simulink model "LGS_allFaultsSelected"  (R2019b)
settings: Solver=FixedStepDiscrete  StartTime=0.0  StopTime=45.0  FixedStep=0.1  RelTol=1e-3
model workspace (MAT data in the model file):
  fipData : object (value not decoded)
  fipName : object (value not decoded)
  stepSize = 0.1
undefined symbols (not defined in the file): ActualSystemCondition, ExpectedSystemBehavior, FailureCondition, FailureConditionObserver, LibFailureCondition
libraries: LibFaultInjectionControls x190, commrandsrc3 x70, simulink x3
(part 15 of 41)

== system LGS_allFaultsSelected/Doors/right door zylinder/sensor open/FIP1 ==
  In1 : Inport
  RD sensor open FIP1 : Subsystem  mask(FailureInjectionPoint){}
      mask help: FailureInjectionPoint
      mask init: same as LGS_allFaultsSelected/Analogical switch and general electro-valve and pressure sensor/Analogical switch/Analog Switch FIP
      settings: OpenFcn=|
      | open_system(gcb,'mask');
      | 
      | treeValues = FailureInjectionPointHelper.getAllFmAndParamsAsTreeString(gcb);
      | mo = Simulink.Mask.get(gcb);
      | dc = mo.getDialogControl('GbFmInfo');
      | treeView = dc.getDialogControl('TreeViewFM');
      | treeView.TreeItems = {};
      | treeView.TreeItems = treeValues;
      mask Help: FailureInjectionPoint
      mask DialogControl Control7 Prompt: Containing Failure Modes
      mask DialogControl BtnMoveUp Prompt: Move up
      mask DialogControl BtnMoveUp Callback:
      | %Get name of the failure mode block
      | mo = Simulink.Mask.get(gcb);
      | dc = mo.getDialogControl('GbFmInfo');
      | treeView = dc.getDialogControl('TreeViewFM');
      | try
      |     a = treeView.getSelectedItems();
      |     p = split(a, '/'); %name of failure mode block is p{1}
      | catch
      |     return;
      | end
      | 
      | %Save port handles
      | lh = get_param([gcb,'/',p{1}],'LineHandles');
      | ph = get_param([gcb,'/',p{1}],'PortHandles');
      | this_in = ph.Inport(1);
      | this_out = ph.Outport(1);
      | 
      | last_block = get_param(lh.Inport(1),'SrcBlockHandle');
      | last_block_type = get_param(last_block,'BlockType');
      | if strcmp(last_block_type,'Inport')
      |     return;
      | end
      | lb_lh = get_param(last_block,'LineHandles');
      | 
      | last_out = get_param(lh.Inport(1),'SrcPortHandle');
      | last_in = get_param(lb_lh.Inport(1),'DstPortHandle');
      | next_to_last_out = get_param(lb_lh.Inport(1),'SrcPortHandle');
      | next_in = get_param(lh.Outport(1),'DstPortHandle');
      | 
      | %Delete connecting lines
      | delete_line(lh.Inport(1));
      | delete_line(lh.Outport(1));
      | delete_line(lb_lh.Inport(1));
      | 
      | % Generate new lines
      | add_line(gcb, last_out, next_in, 'autorouting', 'smart');
      | add_line(gcb, this_out, last_in, 'autorouting', 'smart');
      | add_line(gcb, next_to_last_out, this_in, 'autorouting', 'smart');
      | 
      | %Rearrange system
      | Simulink.BlockDiagram.arrangeSystem(gcb);
      | 
      | %Refresh
      | treeValues = FailureInjectionPointHelper.getAllFmAndParamsAsTreeString(gcb);
      | mo = Simulink.Mask.get(gcb);
      | dc = mo.getDialogControl('GbFmInfo');
      | treeView = dc.getDialogControl('TreeViewFM');
      | treeView.TreeItems = {};
      | treeView.TreeItems = treeValues;
      mask DialogControl BtnMoveDown Prompt: Move down
      mask DialogControl BtnMoveDown Callback:
      | %Get name of the failure mode block
      | mo = Simulink.Mask.get(gcb);
      | dc = mo.getDialogControl('GbFmInfo');
      | treeView = dc.getDialogControl('TreeViewFM');
      | try
      |     a = treeView.getSelectedItems();
      |     p = split(a, '/'); %name of failure mode block is p{1}
      | catch
      |     return;
      | end
      | 
      | %Save port handles
      | lh = get_param([gcb,'/',p{1}],'LineHandles');
      | ph = get_param([gcb,'/',p{1}],'PortHandles');
      | this_in = ph.Inport(1);
      | this_out = ph.Outport(1);
      | 
      | next_block = get_param(lh.Outport(1),'DstBlockHandle');
      | next_block_type = get_param(next_block,'BlockType');
      | if strcmp(next_block_type,'Outport')
      |     return;
      | end
      | nb_lh = get_param(next_block,'LineHandles');
      | 
      | last_out = get_param(lh.Inport(1),'SrcPortHandle');
      | next_out = get_param(nb_lh.Outport(1),'SrcPortHandle');
      | next_but_one_in = get_param(nb_lh.Outport(1),'DstPortHandle');
      | next_in = get_param(lh.Outport(1),'DstPortHandle');
      | 
      | %Delete connecting lines
      | delete_line(lh.Inport(1));
      | delete_line(lh.Outport(1));
      | delete_line(nb_lh.Outport(1));
      | 
      | % Generate new lines
      | add_line(gcb, last_out, next_in, 'autorouting', 'smart');
      | add_line(gcb, next_out, this_in, 'autorouting', 'smart');
      | add_line(gcb, this_out, next_but_one_in, 'autorouting', 'smart');
      | 
      | %Rearrange system
      | Simulink.BlockDiagram.arrangeSystem(gcb);
      | 
      | %Refresh
      | treeValues = FailureInjectionPointHelper.getAllFmAndParamsAsTreeString(gcb);
      | mo = Simulink.Mask.get(gcb);
      | dc = mo.getDialogControl('GbFmInfo');
      | treeView = dc.getDialogControl('TreeViewFM');
      | treeView.TreeItems = {};
      | treeView.TreeItems = treeValues;
      mask DialogControl TreeViewFM Prompt: Failure Mode Information
      mask DialogControl BtnOpen Prompt: Open FIP
      mask DialogControl BtnOpen Callback: open_system(gcb,'force');
      mask DialogControl BtnNew Prompt: New
      mask DialogControl BtnNew Callback:
      | dialog_fipManager_single(gcb, '');
      | 
      | %Enable move, edit, delete buttons
      | mo = Simulink.Mask.get(gcb);
      | mo.getDialogControl('BtnMoveUp').Enabled = 'on';
      | mo.getDialogControl('BtnMoveDown').Enabled = 'on';
      | mo.getDialogControl('BtnEdit').Enabled = 'on';
      | mo.getDialogControl('BtnDelete').Enabled = 'on';
      mask DialogControl BtnEdit Prompt: Edit
      mask DialogControl BtnEdit Callback:
      | mo = Simulink.Mask.get(gcb);
      | dc = mo.getDialogControl('GbFmInfo');
      | treeView = dc.getDialogControl('TreeViewFM');
      | try
      |     a = treeView.getSelectedItems();
      |     p = split(a, '/');
      | catch
      |     return;
      | end
      | dialog_fipManager_single(gcb, p{1});
      mask DialogControl BtnDelete Prompt: Delete
      mask DialogControl BtnDelete Callback:
      | %Get name of the failure mode block
      | mo = Simulink.Mask.get(gcb);
      | dc = mo.getDialogControl('GbFmInfo');
      | treeView = dc.getDialogControl('TreeViewFM');
      | try
      |     a = treeView.getSelectedItems();
      |     p = split(a, '/'); %name of failure mode block is p{1}
      | catch
      |     return;
      | end
      | 
      | %Save outport handle of the last and inport handle of the next block
      | lh = get_param([gcb,'/',p{1}],'LineHandles');
      | last_out = get_param(lh.Inport(1),'SrcPortHandle');
      | next_in = get_param(lh.Outport(1),'DstPortHandle');
      | 
      | %Delete connecting lines and failure mode block
      | delete_line(lh.Inport(1));
      | delete_line(lh.Outport(1));
      | fm_handle = get_param([gcb,'/',p{1}],'Handle');
      | delete_block(fm_handle);
      | 
      | % Generate new line from outport last to inport next
      | add_line(gcb, last_out, next_in, 'autorouting', 'smart');
      | 
      | %Rearrange system
      | Simulink.BlockDiagram.arrangeSystem(gcb);
      | 
      | %Disable move, edit, delete buttons in case all FMs are deleted
      | last_block = get_param(last_out,'Parent');
      | last_is_inport = strcmp(get_param(last_block,'BlockType'),'Inport');
      | next_block = get_param(next_in,'Parent');
      | next_is_outport = strcmp(get_param(next_block,'BlockType'),'Outport');
      | if (last_is_inport && next_is_outport)
      |     mo.getDialogControl('BtnMoveUp').Enabled = 'off';
      |     mo.getDialogControl('BtnMoveDown').Enabled = 'off';
      |     mo.getDialogControl('BtnEdit').Enabled = 'off';
      |     mo.getDialogControl('BtnDelete').Enabled = 'off';
      | end
      | 
      | %Refresh
      | treeValues = FailureInjectionPointHelper.getAllFmAndParamsAsTreeString(gcb);
      | mo = Simulink.Mask.get(gcb);
      | dc = mo.getDialogControl('GbFmInfo');
      | treeView = dc.getDialogControl('TreeViewFM');
      | treeView.TreeItems = {};
      | treeView.TreeItems = treeValues;
      mask DialogControl BtnRefresh Prompt: Refresh
      mask DialogControl BtnRefresh Callback:
      | set_param(gcb,'LinkStatus','none');
      | 
      | treeValues = FailureInjectionPointHelper.getAllFmAndParamsAsTreeString(gcb);
      | mo = Simulink.Mask.get(gcb);
      | dc = mo.getDialogControl('GbFmInfo');
      | treeView = dc.getDialogControl('TreeViewFM');
      | treeView.TreeItems = {};
      | treeView.TreeItems = treeValues;
      mask Display: image('icons/failure_injection_point.png','center')
  Out1 : Outport
  wires:
  In1/1 -> RD sensor open FIP1/1(In1)
  RD sensor open FIP1/1(Out1) -> Out1/1

== system LGS_allFaultsSelected/Doors/right door zylinder/sensor open/FIP2 ==
  In1 : Inport
  RD sensor open FIP2 : Subsystem  mask(FailureInjectionPoint){}
      mask help: FailureInjectionPoint
      mask init: same as LGS_allFaultsSelected/Analogical switch and general electro-valve and pressure sensor/Analogical switch/Analog Switch FIP
      settings: OpenFcn=|
      | open_system(gcb,'mask');
      | 
      | treeValues = FailureInjectionPointHelper.getAllFmAndParamsAsTreeString(gcb);
      | mo = Simulink.Mask.get(gcb);
      | dc = mo.getDialogControl('GbFmInfo');
      | treeView = dc.getDialogControl('TreeViewFM');
      | treeView.TreeItems = {};
      | treeView.TreeItems = treeValues;
      mask Help: FailureInjectionPoint
      mask DialogControl Control7 Prompt: Containing Failure Modes
      mask DialogControl BtnMoveUp Prompt: Move up
      mask DialogControl BtnMoveUp Callback:
      | %Get name of the failure mode block
      | mo = Simulink.Mask.get(gcb);
      | dc = mo.getDialogControl('GbFmInfo');
      | treeView = dc.getDialogControl('TreeViewFM');
      | try
      |     a = treeView.getSelectedItems();
      |     p = split(a, '/'); %name of failure mode block is p{1}
      | catch
      |     return;
      | end
      | 
      | %Save port handles
      | lh = get_param([gcb,'/',p{1}],'LineHandles');
      | ph = get_param([gcb,'/',p{1}],'PortHandles');
      | this_in = ph.Inport(1);
      | this_out = ph.Outport(1);
      | 
      | last_block = get_param(lh.Inport(1),'SrcBlockHandle');
      | last_block_type = get_param(last_block,'BlockType');
      | if strcmp(last_block_type,'Inport')
      |     return;
      | end
      | lb_lh = get_param(last_block,'LineHandles');
      | 
      | last_out = get_param(lh.Inport(1),'SrcPortHandle');
      | last_in = get_param(lb_lh.Inport(1),'DstPortHandle');
      | next_to_last_out = get_param(lb_lh.Inport(1),'SrcPortHandle');
      | next_in = get_param(lh.Outport(1),'DstPortHandle');
      | 
      | %Delete connecting lines
      | delete_line(lh.Inport(1));
      | delete_line(lh.Outport(1));
      | delete_line(lb_lh.Inport(1));
      | 
      | % Generate new lines
      | add_line(gcb, last_out, next_in, 'autorouting', 'smart');
      | add_line(gcb, this_out, last_in, 'autorouting', 'smart');
      | add_line(gcb, next_to_last_out, this_in, 'autorouting', 'smart');
      | 
      | %Rearrange system
      | Simulink.BlockDiagram.arrangeSystem(gcb);
      | 
      | %Refresh
      | treeValues = FailureInjectionPointHelper.getAllFmAndParamsAsTreeString(gcb);
      | mo = Simulink.Mask.get(gcb);
      | dc = mo.getDialogControl('GbFmInfo');
      | treeView = dc.getDialogControl('TreeViewFM');
      | treeView.TreeItems = {};
      | treeView.TreeItems = treeValues;
      mask DialogControl BtnMoveDown Prompt: Move down
      mask DialogControl BtnMoveDown Callback:
      | %Get name of the failure mode block
      | mo = Simulink.Mask.get(gcb);
      | dc = mo.getDialogControl('GbFmInfo');
      | treeView = dc.getDialogControl('TreeViewFM');
      | try
      |     a = treeView.getSelectedItems();
      |     p = split(a, '/'); %name of failure mode block is p{1}
      | catch
      |     return;
      | end
      | 
      | %Save port handles
      | lh = get_param([gcb,'/',p{1}],'LineHandles');
      | ph = get_param([gcb,'/',p{1}],'PortHandles');
      | this_in = ph.Inport(1);
      | this_out = ph.Outport(1);
      | 
      | next_block = get_param(lh.Outport(1),'DstBlockHandle');
      | next_block_type = get_param(next_block,'BlockType');
      | if strcmp(next_block_type,'Outport')
      |     return;
      | end
      | nb_lh = get_param(next_block,'LineHandles');
      | 
      | last_out = get_param(lh.Inport(1),'SrcPortHandle');
      | next_out = get_param(nb_lh.Outport(1),'SrcPortHandle');
      | next_but_one_in = get_param(nb_lh.Outport(1),'DstPortHandle');
      | next_in = get_param(lh.Outport(1),'DstPortHandle');
      | 
      | %Delete connecting lines
      | delete_line(lh.Inport(1));
      | delete_line(lh.Outport(1));
      | delete_line(nb_lh.Outport(1));
      | 
      | % Generate new lines
      | add_line(gcb, last_out, next_in, 'autorouting', 'smart');
      | add_line(gcb, next_out, this_in, 'autorouting', 'smart');
      | add_line(gcb, this_out, next_but_one_in, 'autorouting', 'smart');
      | 
      | %Rearrange system
      | Simulink.BlockDiagram.arrangeSystem(gcb);
      | 
      | %Refresh
      | treeValues = FailureInjectionPointHelper.getAllFmAndParamsAsTreeString(gcb);
      | mo = Simulink.Mask.get(gcb);
      | dc = mo.getDialogControl('GbFmInfo');
      | treeView = dc.getDialogControl('TreeViewFM');
      | treeView.TreeItems = {};
      | treeView.TreeItems = treeValues;
      mask DialogControl TreeViewFM Prompt: Failure Mode Information
      mask DialogControl BtnOpen Prompt: Open FIP
      mask DialogControl BtnOpen Callback: open_system(gcb,'force');
      mask DialogControl BtnNew Prompt: New
      mask DialogControl BtnNew Callback:
      | dialog_fipManager_single(gcb, '');
      | 
      | %Enable move, edit, delete buttons
      | mo = Simulink.Mask.get(gcb);
      | mo.getDialogControl('BtnMoveUp').Enabled = 'on';
      | mo.getDialogControl('BtnMoveDown').Enabled = 'on';
      | mo.getDialogControl('BtnEdit').Enabled = 'on';
      | mo.getDialogControl('BtnDelete').Enabled = 'on';
      mask DialogControl BtnEdit Prompt: Edit
      mask DialogControl BtnEdit Callback:
      | mo = Simulink.Mask.get(gcb);
      | dc = mo.getDialogControl('GbFmInfo');
      | treeView = dc.getDialogControl('TreeViewFM');
      | try
      |     a = treeView.getSelectedItems();
      |     p = split(a, '/');
      | catch
      |     return;
      | end
      | dialog_fipManager_single(gcb, p{1});
      mask DialogControl BtnDelete Prompt: Delete
      mask DialogControl BtnDelete Callback:
      | %Get name of the failure mode block
      | mo = Simulink.Mask.get(gcb);
      | dc = mo.getDialogControl('GbFmInfo');
      | treeView = dc.getDialogControl('TreeViewFM');
      | try
      |     a = treeView.getSelectedItems();
      |     p = split(a, '/'); %name of failure mode block is p{1}
      | catch
      |     return;
      | end
      | 
      | %Save outport handle of the last and inport handle of the next block
      | lh = get_param([gcb,'/',p{1}],'LineHandles');
      | last_out = get_param(lh.Inport(1),'SrcPortHandle');
      | next_in = get_param(lh.Outport(1),'DstPortHandle');
      | 
      | %Delete connecting lines and failure mode block
      | delete_line(lh.Inport(1));
      | delete_line(lh.Outport(1));
      | fm_handle = get_param([gcb,'/',p{1}],'Handle');
      | delete_block(fm_handle);
      | 
      | % Generate new line from outport last to inport next
      | add_line(gcb, last_out, next_in, 'autorouting', 'smart');
      | 
      | %Rearrange system
      | Simulink.BlockDiagram.arrangeSystem(gcb);
      | 
      | %Disable move, edit, delete buttons in case all FMs are deleted
      | last_block = get_param(last_out,'Parent');
      | last_is_inport = strcmp(get_param(last_block,'BlockType'),'Inport');
      | next_block = get_param(next_in,'Parent');
      | next_is_outport = strcmp(get_param(next_block,'BlockType'),'Outport');
      | if (last_is_inport && next_is_outport)
      |     mo.getDialogControl('BtnMoveUp').Enabled = 'off';
      |     mo.getDialogControl('BtnMoveDown').Enabled = 'off';
      |     mo.getDialogControl('BtnEdit').Enabled = 'off';
      |     mo.getDialogControl('BtnDelete').Enabled = 'off';
      | end
      | 
      | %Refresh
      | treeValues = FailureInjectionPointHelper.getAllFmAndParamsAsTreeString(gcb);
      | mo = Simulink.Mask.get(gcb);
      | dc = mo.getDialogControl('GbFmInfo');
      | treeView = dc.getDialogControl('TreeViewFM');
      | treeView.TreeItems = {};
      | treeView.TreeItems = treeValues;
      mask DialogControl BtnRefresh Prompt: Refresh
      mask DialogControl BtnRefresh Callback:
      | set_param(gcb,'LinkStatus','none');
      | 
      | treeValues = FailureInjectionPointHelper.getAllFmAndParamsAsTreeString(gcb);
      | mo = Simulink.Mask.get(gcb);
      | dc = mo.getDialogControl('GbFmInfo');
      | treeView = dc.getDialogControl('TreeViewFM');
      | treeView.TreeItems = {};
      | treeView.TreeItems = treeValues;
      mask Display: image('icons/failure_injection_point.png','center')
  Out1 : Outport
  wires:
  In1/1 -> RD sensor open FIP2/1(In1)
  RD sensor open FIP2/1(Out1) -> Out1/1

== system LGS_allFaultsSelected/Doors/right door zylinder/sensor open/FIP3 ==
  In1 : Inport
  RD sensor open FIP3 : Subsystem  mask(FailureInjectionPoint){}
      mask help: FailureInjectionPoint
      mask init: same as LGS_allFaultsSelected/Analogical switch and general electro-valve and pressure sensor/Analogical switch/Analog Switch FIP
      settings: OpenFcn=|
      | open_system(gcb,'mask');
      | 
      | treeValues = FailureInjectionPointHelper.getAllFmAndParamsAsTreeString(gcb);
      | mo = Simulink.Mask.get(gcb);
      | dc = mo.getDialogControl('GbFmInfo');
      | treeView = dc.getDialogControl('TreeViewFM');
      | treeView.TreeItems = {};
      | treeView.TreeItems = treeValues;
      mask Help: FailureInjectionPoint
      mask DialogControl Control7 Prompt: Containing Failure Modes
      mask DialogControl BtnMoveUp Prompt: Move up
      mask DialogControl BtnMoveUp Callback:
      | %Get name of the failure mode block
      | mo = Simulink.Mask.get(gcb);
      | dc = mo.getDialogControl('GbFmInfo');
      | treeView = dc.getDialogControl('TreeViewFM');
      | try
      |     a = treeView.getSelectedItems();
      |     p = split(a, '/'); %name of failure mode block is p{1}
      | catch
      |     return;
      | end
      | 
      | %Save port handles
      | lh = get_param([gcb,'/',p{1}],'LineHandles');
      | ph = get_param([gcb,'/',p{1}],'PortHandles');
      | this_in = ph.Inport(1);
      | this_out = ph.Outport(1);
      | 
      | last_block = get_param(lh.Inport(1),'SrcBlockHandle');
      | last_block_type = get_param(last_block,'BlockType');
      | if strcmp(last_block_type,'Inport')
      |     return;
      | end
      | lb_lh = get_param(last_block,'LineHandles');
      | 
      | last_out = get_param(lh.Inport(1),'SrcPortHandle');
      | last_in = get_param(lb_lh.Inport(1),'DstPortHandle');
      | next_to_last_out = get_param(lb_lh.Inport(1),'SrcPortHandle');
      | next_in = get_param(lh.Outport(1),'DstPortHandle');
      | 
      | %Delete connecting lines
      | delete_line(lh.Inport(1));
      | delete_line(lh.Outport(1));
      | delete_line(lb_lh.Inport(1));
      | 
      | % Generate new lines
      | add_line(gcb, last_out, next_in, 'autorouting', 'smart');
      | add_line(gcb, this_out, last_in, 'autorouting', 'smart');
      | add_line(gcb, next_to_last_out, this_in, 'autorouting', 'smart');
      | 
      | %Rearrange system
      | Simulink.BlockDiagram.arrangeSystem(gcb);
      | 
      | %Refresh
      | treeValues = FailureInjectionPointHelper.getAllFmAndParamsAsTreeString(gcb);
      | mo = Simulink.Mask.get(gcb);
      | dc = mo.getDialogControl('GbFmInfo');
      | treeView = dc.getDialogControl('TreeViewFM');
      | treeView.TreeItems = {};
      | treeView.TreeItems = treeValues;
      mask DialogControl BtnMoveDown Prompt: Move down
      mask DialogControl BtnMoveDown Callback:
      | %Get name of the failure mode block
      | mo = Simulink.Mask.get(gcb);
      | dc = mo.getDialogControl('GbFmInfo');
      | treeView = dc.getDialogControl('TreeViewFM');
      | try
      |     a = treeView.getSelectedItems();
      |     p = split(a, '/'); %name of failure mode block is p{1}
      | catch
      |     return;
      | end
      | 
      | %Save port handles
      | lh = get_param([gcb,'/',p{1}],'LineHandles');
      | ph = get_param([gcb,'/',p{1}],'PortHandles');
      | this_in = ph.Inport(1);
      | this_out = ph.Outport(1);
      | 
      | next_block = get_param(lh.Outport(1),'DstBlockHandle');
      | next_block_type = get_param(next_block,'BlockType');
      | if strcmp(next_block_type,'Outport')
      |     return;
      | end
      | nb_lh = get_param(next_block,'LineHandles');
      | 
      | last_out = get_param(lh.Inport(1),'SrcPortHandle');
      | next_out = get_param(nb_lh.Outport(1),'SrcPortHandle');
      | next_but_one_in = get_param(nb_lh.Outport(1),'DstPortHandle');
      | next_in = get_param(lh.Outport(1),'DstPortHandle');
      | 
      | %Delete connecting lines
      | delete_line(lh.Inport(1));
      | delete_line(lh.Outport(1));
      | delete_line(nb_lh.Outport(1));
      | 
      | % Generate new lines
      | add_line(gcb, last_out, next_in, 'autorouting', 'smart');
      | add_line(gcb, next_out, this_in, 'autorouting', 'smart');
      | add_line(gcb, this_out, next_but_one_in, 'autorouting', 'smart');
      | 
      | %Rearrange system
      | Simulink.BlockDiagram.arrangeSystem(gcb);
      | 
      | %Refresh
      | treeValues = FailureInjectionPointHelper.getAllFmAndParamsAsTreeString(gcb);
      | mo = Simulink.Mask.get(gcb);
      | dc = mo.getDialogControl('GbFmInfo');
      | treeView = dc.getDialogControl('TreeViewFM');
      | treeView.TreeItems = {};
      | treeView.TreeItems = treeValues;
      mask DialogControl TreeViewFM Prompt: Failure Mode Information
      mask DialogControl BtnOpen Prompt: Open FIP
      mask DialogControl BtnOpen Callback: open_system(gcb,'force');
      mask DialogControl BtnNew Prompt: New
      mask DialogControl BtnNew Callback:
      | dialog_fipManager_single(gcb, '');
      | 
      | %Enable move, edit, delete buttons
      | mo = Simulink.Mask.get(gcb);
      | mo.getDialogControl('BtnMoveUp').Enabled = 'on';
      | mo.getDialogControl('BtnMoveDown').Enabled = 'on';
      | mo.getDialogControl('BtnEdit').Enabled = 'on';
      | mo.getDialogControl('BtnDelete').Enabled = 'on';
      mask DialogControl BtnEdit Prompt: Edit
      mask DialogControl BtnEdit Callback:
      | mo = Simulink.Mask.get(gcb);
      | dc = mo.getDialogControl('GbFmInfo');
      | treeView = dc.getDialogControl('TreeViewFM');
      | try
      |     a = treeView.getSelectedItems();
      |     p = split(a, '/');
      | catch
      |     return;
      | end
      | dialog_fipManager_single(gcb, p{1});
      mask DialogControl BtnDelete Prompt: Delete
      mask DialogControl BtnDelete Callback:
      | %Get name of the failure mode block
      | mo = Simulink.Mask.get(gcb);
      | dc = mo.getDialogControl('GbFmInfo');
      | treeView = dc.getDialogControl('TreeViewFM');
      | try
      |     a = treeView.getSelectedItems();
      |     p = split(a, '/'); %name of failure mode block is p{1}
      | catch
      |     return;
      | end
      | 
      | %Save outport handle of the last and inport handle of the next block
      | lh = get_param([gcb,'/',p{1}],'LineHandles');
      | last_out = get_param(lh.Inport(1),'SrcPortHandle');
      | next_in = get_param(lh.Outport(1),'DstPortHandle');
      | 
      | %Delete connecting lines and failure mode block
      | delete_line(lh.Inport(1));
      | delete_line(lh.Outport(1));
      | fm_handle = get_param([gcb,'/',p{1}],'Handle');
      | delete_block(fm_handle);
      | 
      | % Generate new line from outport last to inport next
      | add_line(gcb, last_out, next_in, 'autorouting', 'smart');
      | 
      | %Rearrange system
      | Simulink.BlockDiagram.arrangeSystem(gcb);
      | 
      | %Disable move, edit, delete buttons in case all FMs are deleted
      | last_block = get_param(last_out,'Parent');
      | last_is_inport = strcmp(get_param(last_block,'BlockType'),'Inport');
      | next_block = get_param(next_in,'Parent');
      | next_is_outport = strcmp(get_param(next_block,'BlockType'),'Outport');
      | if (last_is_inport && next_is_outport)
      |     mo.getDialogControl('BtnMoveUp').Enabled = 'off';
      |     mo.getDialogControl('BtnMoveDown').Enabled = 'off';
      |     mo.getDialogControl('BtnEdit').Enabled = 'off';
      |     mo.getDialogControl('BtnDelete').Enabled = 'off';
      | end
      | 
      | %Refresh
      | treeValues = FailureInjectionPointHelper.getAllFmAndParamsAsTreeString(gcb);
      | mo = Simulink.Mask.get(gcb);
      | dc = mo.getDialogControl('GbFmInfo');
      | treeView = dc.getDialogControl('TreeViewFM');
      | treeView.TreeItems = {};
      | treeView.TreeItems = treeValues;
      mask DialogControl BtnRefresh Prompt: Refresh
      mask DialogControl BtnRefresh Callback:
      | set_param(gcb,'LinkStatus','none');
      | 
      | treeValues = FailureInjectionPointHelper.getAllFmAndParamsAsTreeString(gcb);
      | mo = Simulink.Mask.get(gcb);
      | dc = mo.getDialogControl('GbFmInfo');
      | treeView = dc.getDialogControl('TreeViewFM');
      | treeView.TreeItems = {};
      | treeView.TreeItems = treeValues;
      mask Display: image('icons/failure_injection_point.png','center')
  Out1 : Outport
  wires:
  In1/1 -> RD sensor open FIP3/1(In1)
  RD sensor open FIP3/1(Out1) -> Out1/1

== system LGS_allFaultsSelected/Gears/EV extend gear/EV extend gear FIP/Blocked closed ==
  In1 : Inport
  CommitValue : Constant  Value=Value  OutDataTypeStr=boolean
  Switch : Switch  Criteria=u2 > Threshold
  Trigger FIP : LibFaultInjectionControls/Trigger FIP  Active=on  MaintenanceTask=MaintenanceTask  RiskTime=RiskTime  FailureRate=FailureRate  isDSF=off  DSFjson=JSON
      settings: SourceProductName=Fault Injection Controls
  Out1 : Outport
  wires:
  In1/1 -> Switch/3
  Trigger FIP/1 -> Switch/2
  Switch/1 -> Out1/1
  CommitValue/1 -> Switch/1

== system LGS_allFaultsSelected/Gears/EV extend gear/EV extend gear FIP/Blocked open ==
  In1 : Inport
  CommitValue : Constant  Value=Value  OutDataTypeStr=boolean
  Switch : Switch  Criteria=u2 > Threshold
  Trigger FIP : LibFaultInjectionControls/Trigger FIP  Active=on  MaintenanceTask=MaintenanceTask  RiskTime=RiskTime  FailureRate=FailureRate  isDSF=off  DSFjson=JSON
      settings: SourceProductName=Fault Injection Controls
  Out1 : Outport
  wires:
  In1/1 -> Switch/3
  Trigger FIP/1 -> Switch/2
  Switch/1 -> Out1/1
  CommitValue/1 -> Switch/1

== system LGS_allFaultsSelected/Gears/EV retract gear/EV retract gear FIP/Blocked closed ==
  In1 : Inport
  CommitValue : Constant  Value=Value  OutDataTypeStr=boolean
  Switch : Switch  Criteria=u2 > Threshold
  Trigger FIP : LibFaultInjectionControls/Trigger FIP  Active=on  MaintenanceTask=MaintenanceTask  RiskTime=RiskTime  FailureRate=FailureRate  isDSF=off  DSFjson=JSON
      settings: SourceProductName=Fault Injection Controls
  Out1 : Outport
  wires:
  In1/1 -> Switch/3
  Trigger FIP/1 -> Switch/2
  Switch/1 -> Out1/1
  CommitValue/1 -> Switch/1

== system LGS_allFaultsSelected/Gears/EV retract gear/EV retract gear FIP/Blocked open ==
  In1 : Inport
  CommitValue : Constant  Value=Value  OutDataTypeStr=boolean
  Switch : Switch  Criteria=u2 > Threshold
  Trigger FIP : LibFaultInjectionControls/Trigger FIP  Active=on  MaintenanceTask=MaintenanceTask  RiskTime=RiskTime  FailureRate=FailureRate  isDSF=off  DSFjson=JSON
      settings: SourceProductName=Fault Injection Controls
  Out1 : Outport
  wires:
  In1/1 -> Switch/3
  Trigger FIP/1 -> Switch/2
  Switch/1 -> Out1/1
  CommitValue/1 -> Switch/1

== system LGS_allFaultsSelected/Gears/FG shock absorber/sensor shock absorber/FIP1 ==
  In1 : Inport
  FG sensor shock absorber FIP1 : Subsystem  mask(FailureInjectionPoint){}
      mask help: FailureInjectionPoint
      mask init: same as LGS_allFaultsSelected/Analogical switch and general electro-valve and pressure sensor/Analogical switch/Analog Switch FIP
      settings: OpenFcn=|
      | open_system(gcb,'mask');
      | 
      | treeValues = FailureInjectionPointHelper.getAllFmAndParamsAsTreeString(gcb);
      | mo = Simulink.Mask.get(gcb);
      | dc = mo.getDialogControl('GbFmInfo');
      | treeView = dc.getDialogControl('TreeViewFM');
      | treeView.TreeItems = {};
      | treeView.TreeItems = treeValues;
      mask Help: FailureInjectionPoint
      mask DialogControl Control7 Prompt: Containing Failure Modes
      mask DialogControl BtnMoveUp Prompt: Move up
      mask DialogControl BtnMoveUp Callback:
      | %Get name of the failure mode block
      | mo = Simulink.Mask.get(gcb);
      | dc = mo.getDialogControl('GbFmInfo');
      | treeView = dc.getDialogControl('TreeViewFM');
      | try
      |     a = treeView.getSelectedItems();
      |     p = split(a, '/'); %name of failure mode block is p{1}
      | catch
      |     return;
      | end
      | 
      | %Save port handles
      | lh = get_param([gcb,'/',p{1}],'LineHandles');
      | ph = get_param([gcb,'/',p{1}],'PortHandles');
      | this_in = ph.Inport(1);
      | this_out = ph.Outport(1);
      | 
      | last_block = get_param(lh.Inport(1),'SrcBlockHandle');
      | last_block_type = get_param(last_block,'BlockType');
      | if strcmp(last_block_type,'Inport')
      |     return;
      | end
      | lb_lh = get_param(last_block,'LineHandles');
      | 
      | last_out = get_param(lh.Inport(1),'SrcPortHandle');
      | last_in = get_param(lb_lh.Inport(1),'DstPortHandle');
      | next_to_last_out = get_param(lb_lh.Inport(1),'SrcPortHandle');
      | next_in = get_param(lh.Outport(1),'DstPortHandle');
      | 
      | %Delete connecting lines
      | delete_line(lh.Inport(1));
      | delete_line(lh.Outport(1));
      | delete_line(lb_lh.Inport(1));
      | 
      | % Generate new lines
      | add_line(gcb, last_out, next_in, 'autorouting', 'smart');
      | add_line(gcb, this_out, last_in, 'autorouting', 'smart');
      | add_line(gcb, next_to_last_out, this_in, 'autorouting', 'smart');
      | 
      | %Rearrange system
      | Simulink.BlockDiagram.arrangeSystem(gcb);
      | 
      | %Refresh
      | treeValues = FailureInjectionPointHelper.getAllFmAndParamsAsTreeString(gcb);
      | mo = Simulink.Mask.get(gcb);
      | dc = mo.getDialogControl('GbFmInfo');
      | treeView = dc.getDialogControl('TreeViewFM');
      | treeView.TreeItems = {};
      | treeView.TreeItems = treeValues;
      mask DialogControl BtnMoveDown Prompt: Move down
      mask DialogControl BtnMoveDown Callback:
      | %Get name of the failure mode block
      | mo = Simulink.Mask.get(gcb);
      | dc = mo.getDialogControl('GbFmInfo');
      | treeView = dc.getDialogControl('TreeViewFM');
      | try
      |     a = treeView.getSelectedItems();
      |     p = split(a, '/'); %name of failure mode block is p{1}
      | catch
      |     return;
      | end
      | 
      | %Save port handles
      | lh = get_param([gcb,'/',p{1}],'LineHandles');
      | ph = get_param([gcb,'/',p{1}],'PortHandles');
      | this_in = ph.Inport(1);
      | this_out = ph.Outport(1);
      | 
      | next_block = get_param(lh.Outport(1),'DstBlockHandle');
      | next_block_type = get_param(next_block,'BlockType');
      | if strcmp(next_block_type,'Outport')
      |     return;
      | end
      | nb_lh = get_param(next_block,'LineHandles');
      | 
      | last_out = get_param(lh.Inport(1),'SrcPortHandle');
      | next_out = get_param(nb_lh.Outport(1),'SrcPortHandle');
      | next_but_one_in = get_param(nb_lh.Outport(1),'DstPortHandle');
      | next_in = get_param(lh.Outport(1),'DstPortHandle');
      | 
      | %Delete connecting lines
      | delete_line(lh.Inport(1));
      | delete_line(lh.Outport(1));
      | delete_line(nb_lh.Outport(1));
      | 
      | % Generate new lines
      | add_line(gcb, last_out, next_in, 'autorouting', 'smart');
      | add_line(gcb, next_out, this_in, 'autorouting', 'smart');
      | add_line(gcb, this_out, next_but_one_in, 'autorouting', 'smart');
      | 
      | %Rearrange system
      | Simulink.BlockDiagram.arrangeSystem(gcb);
      | 
      | %Refresh
      | treeValues = FailureInjectionPointHelper.getAllFmAndParamsAsTreeString(gcb);
      | mo = Simulink.Mask.get(gcb);
      | dc = mo.getDialogControl('GbFmInfo');
      | treeView = dc.getDialogControl('TreeViewFM');
      | treeView.TreeItems = {};
      | treeView.TreeItems = treeValues;
      mask DialogControl TreeViewFM Prompt: Failure Mode Information
      mask DialogControl BtnOpen Prompt: Open FIP
      mask DialogControl BtnOpen Callback: open_system(gcb,'force');
      mask DialogControl BtnNew Prompt: New
      mask DialogControl BtnNew Callback:
      | dialog_fipManager_single(gcb, '');
      | 
      | %Enable move, edit, delete buttons
      | mo = Simulink.Mask.get(gcb);
      | mo.getDialogControl('BtnMoveUp').Enabled = 'on';
      | mo.getDialogControl('BtnMoveDown').Enabled = 'on';
      | mo.getDialogControl('BtnEdit').Enabled = 'on';
      | mo.getDialogControl('BtnDelete').Enabled = 'on';
      mask DialogControl BtnEdit Prompt: Edit
      mask DialogControl BtnEdit Callback:
      | mo = Simulink.Mask.get(gcb);
      | dc = mo.getDialogControl('GbFmInfo');
      | treeView = dc.getDialogControl('TreeViewFM');
      | try
      |     a = treeView.getSelectedItems();
      |     p = split(a, '/');
      | catch
      |     return;
      | end
      | dialog_fipManager_single(gcb, p{1});
      mask DialogControl BtnDelete Prompt: Delete
      mask DialogControl BtnDelete Callback:
      | %Get name of the failure mode block
      | mo = Simulink.Mask.get(gcb);
      | dc = mo.getDialogControl('GbFmInfo');
      | treeView = dc.getDialogControl('TreeViewFM');
      | try
      |     a = treeView.getSelectedItems();
      |     p = split(a, '/'); %name of failure mode block is p{1}
      | catch
      |     return;
      | end
      | 
      | %Save outport handle of the last and inport handle of the next block
      | lh = get_param([gcb,'/',p{1}],'LineHandles');
      | last_out = get_param(lh.Inport(1),'SrcPortHandle');
      | next_in = get_param(lh.Outport(1),'DstPortHandle');
      | 
      | %Delete connecting lines and failure mode block
      | delete_line(lh.Inport(1));
      | delete_line(lh.Outport(1));
      | fm_handle = get_param([gcb,'/',p{1}],'Handle');
      | delete_block(fm_handle);
      | 
      | % Generate new line from outport last to inport next
      | add_line(gcb, last_out, next_in, 'autorouting', 'smart');
      | 
      | %Rearrange system
      | Simulink.BlockDiagram.arrangeSystem(gcb);
      | 
      | %Disable move, edit, delete buttons in case all FMs are deleted
      | last_block = get_param(last_out,'Parent');
      | last_is_inport = strcmp(get_param(last_block,'BlockType'),'Inport');
      | next_block = get_param(next_in,'Parent');
      | next_is_outport = strcmp(get_param(next_block,'BlockType'),'Outport');
      | if (last_is_inport && next_is_outport)
      |     mo.getDialogControl('BtnMoveUp').Enabled = 'off';
      |     mo.getDialogControl('BtnMoveDown').Enabled = 'off';
      |     mo.getDialogControl('BtnEdit').Enabled = 'off';
      |     mo.getDialogControl('BtnDelete').Enabled = 'off';
      | end
      | 
      | %Refresh
      | treeValues = FailureInjectionPointHelper.getAllFmAndParamsAsTreeString(gcb);
      | mo = Simulink.Mask.get(gcb);
      | dc = mo.getDialogControl('GbFmInfo');
      | treeView = dc.getDialogControl('TreeViewFM');
      | treeView.TreeItems = {};
      | treeView.TreeItems = treeValues;
      mask DialogControl BtnRefresh Prompt: Refresh
      mask DialogControl BtnRefresh Callback:
      | set_param(gcb,'LinkStatus','none');
      | 
      | treeValues = FailureInjectionPointHelper.getAllFmAndParamsAsTreeString(gcb);
      | mo = Simulink.Mask.get(gcb);
      | dc = mo.getDialogControl('GbFmInfo');
      | treeView = dc.getDialogControl('TreeViewFM');
      | treeView.TreeItems = {};
      | treeView.TreeItems = treeValues;
      mask Display: image('icons/failure_injection_point.png','center')
  Out1 : Outport
  wires:
  In1/1 -> FG sensor shock absorber FIP1/1(In1)
  FG sensor shock absorber FIP1/1(Out1) -> Out1/1

== system LGS_allFaultsSelected/Gears/FG shock absorber/sensor shock absorber/FIP2 ==
  In1 : Inport
  FG sensor shock absorber FIP2 : Subsystem  mask(FailureInjectionPoint){}
      mask help: FailureInjectionPoint
      mask init: same as LGS_allFaultsSelected/Analogical switch and general electro-valve and pressure sensor/Analogical switch/Analog Switch FIP
      settings: OpenFcn=|
      | open_system(gcb,'mask');
      | 
      | treeValues = FailureInjectionPointHelper.getAllFmAndParamsAsTreeString(gcb);
      | mo = Simulink.Mask.get(gcb);
      | dc = mo.getDialogControl('GbFmInfo');
      | treeView = dc.getDialogControl('TreeViewFM');
      | treeView.TreeItems = {};
      | treeView.TreeItems = treeValues;
      mask Help: FailureInjectionPoint
      mask DialogControl Control7 Prompt: Containing Failure Modes
      mask DialogControl BtnMoveUp Prompt: Move up
      mask DialogControl BtnMoveUp Callback:
      | %Get name of the failure mode block
      | mo = Simulink.Mask.get(gcb);
      | dc = mo.getDialogControl('GbFmInfo');
      | treeView = dc.getDialogControl('TreeViewFM');
      | try
      |     a = treeView.getSelectedItems();
      |     p = split(a, '/'); %name of failure mode block is p{1}
      | catch
      |     return;
      | end
      | 
      | %Save port handles
      | lh = get_param([gcb,'/',p{1}],'LineHandles');
      | ph = get_param([gcb,'/',p{1}],'PortHandles');
      | this_in = ph.Inport(1);
      | this_out = ph.Outport(1);
      | 
      | last_block = get_param(lh.Inport(1),'SrcBlockHandle');
      | last_block_type = get_param(last_block,'BlockType');
      | if strcmp(last_block_type,'Inport')
      |     return;
      | end
      | lb_lh = get_param(last_block,'LineHandles');
      | 
      | last_out = get_param(lh.Inport(1),'SrcPortHandle');
      | last_in = get_param(lb_lh.Inport(1),'DstPortHandle');
      | next_to_last_out = get_param(lb_lh.Inport(1),'SrcPortHandle');
      | next_in = get_param(lh.Outport(1),'DstPortHandle');
      | 
      | %Delete connecting lines
      | delete_line(lh.Inport(1));
      | delete_line(lh.Outport(1));
      | delete_line(lb_lh.Inport(1));
      | 
      | % Generate new lines
      | add_line(gcb, last_out, next_in, 'autorouting', 'smart');
      | add_line(gcb, this_out, last_in, 'autorouting', 'smart');
      | add_line(gcb, next_to_last_out, this_in, 'autorouting', 'smart');
      | 
      | %Rearrange system
      | Simulink.BlockDiagram.arrangeSystem(gcb);
      | 
      | %Refresh
      | treeValues = FailureInjectionPointHelper.getAllFmAndParamsAsTreeString(gcb);
      | mo = Simulink.Mask.get(gcb);
      | dc = mo.getDialogControl('GbFmInfo');
      | treeView = dc.getDialogControl('TreeViewFM');
      | treeView.TreeItems = {};
      | treeView.TreeItems = treeValues;
      mask DialogControl BtnMoveDown Prompt: Move down
      mask DialogControl BtnMoveDown Callback:
      | %Get name of the failure mode block
      | mo = Simulink.Mask.get(gcb);
      | dc = mo.getDialogControl('GbFmInfo');
      | treeView = dc.getDialogControl('TreeViewFM');
      | try
      |     a = treeView.getSelectedItems();
      |     p = split(a, '/'); %name of failure mode block is p{1}
      | catch
      |     return;
      | end
      | 
      | %Save port handles
      | lh = get_param([gcb,'/',p{1}],'LineHandles');
      | ph = get_param([gcb,'/',p{1}],'PortHandles');
      | this_in = ph.Inport(1);
      | this_out = ph.Outport(1);
      | 
      | next_block = get_param(lh.Outport(1),'DstBlockHandle');
      | next_block_type = get_param(next_block,'BlockType');
      | if strcmp(next_block_type,'Outport')
      |     return;
      | end
      | nb_lh = get_param(next_block,'LineHandles');
      | 
      | last_out = get_param(lh.Inport(1),'SrcPortHandle');
      | next_out = get_param(nb_lh.Outport(1),'SrcPortHandle');
      | next_but_one_in = get_param(nb_lh.Outport(1),'DstPortHandle');
      | next_in = get_param(lh.Outport(1),'DstPortHandle');
      | 
      | %Delete connecting lines
      | delete_line(lh.Inport(1));
      | delete_line(lh.Outport(1));
      | delete_line(nb_lh.Outport(1));
      | 
      | % Generate new lines
      | add_line(gcb, last_out, next_in, 'autorouting', 'smart');
      | add_line(gcb, next_out, this_in, 'autorouting', 'smart');
      | add_line(gcb, this_out, next_but_one_in, 'autorouting', 'smart');
      | 
      | %Rearrange system
      | Simulink.BlockDiagram.arrangeSystem(gcb);
      | 
      | %Refresh
      | treeValues = FailureInjectionPointHelper.getAllFmAndParamsAsTreeString(gcb);
      | mo = Simulink.Mask.get(gcb);
      | dc = mo.getDialogControl('GbFmInfo');
      | treeView = dc.getDialogControl('TreeViewFM');
      | treeView.TreeItems = {};
      | treeView.TreeItems = treeValues;
      mask DialogControl TreeViewFM Prompt: Failure Mode Information
      mask DialogControl BtnOpen Prompt: Open FIP
      mask DialogControl BtnOpen Callback: open_system(gcb,'force');
      mask DialogControl BtnNew Prompt: New
      mask DialogControl BtnNew Callback:
      | dialog_fipManager_single(gcb, '');
      | 
      | %Enable move, edit, delete buttons
      | mo = Simulink.Mask.get(gcb);
      | mo.getDialogControl('BtnMoveUp').Enabled = 'on';
      | mo.getDialogControl('BtnMoveDown').Enabled = 'on';
      | mo.getDialogControl('BtnEdit').Enabled = 'on';
      | mo.getDialogControl('BtnDelete').Enabled = 'on';
      mask DialogControl BtnEdit Prompt: Edit
      mask DialogControl BtnEdit Callback:
      | mo = Simulink.Mask.get(gcb);
      | dc = mo.getDialogControl('GbFmInfo');
      | treeView = dc.getDialogControl('TreeViewFM');
      | try
      |     a = treeView.getSelectedItems();
      |     p = split(a, '/');
      | catch
      |     return;
      | end
      | dialog_fipManager_single(gcb, p{1});
      mask DialogControl BtnDelete Prompt: Delete
      mask DialogControl BtnDelete Callback:
      | %Get name of the failure mode block
      | mo = Simulink.Mask.get(gcb);
      | dc = mo.getDialogControl('GbFmInfo');
      | treeView = dc.getDialogControl('TreeViewFM');
      | try
      |     a = treeView.getSelectedItems();
      |     p = split(a, '/'); %name of failure mode block is p{1}
      | catch
      |     return;
      | end
      | 
      | %Save outport handle of the last and inport handle of the next block
      | lh = get_param([gcb,'/',p{1}],'LineHandles');
      | last_out = get_param(lh.Inport(1),'SrcPortHandle');
      | next_in = get_param(lh.Outport(1),'DstPortHandle');
      | 
      | %Delete connecting lines and failure mode block
      | delete_line(lh.Inport(1));
      | delete_line(lh.Outport(1));
      | fm_handle = get_param([gcb,'/',p{1}],'Handle');
      | delete_block(fm_handle);
      | 
      | % Generate new line from outport last to inport next
      | add_line(gcb, last_out, next_in, 'autorouting', 'smart');
      | 
      | %Rearrange system
      | Simulink.BlockDiagram.arrangeSystem(gcb);
      | 
      | %Disable move, edit, delete buttons in case all FMs are deleted
      | last_block = get_param(last_out,'Parent');
      | last_is_inport = strcmp(get_param(last_block,'BlockType'),'Inport');
      | next_block = get_param(next_in,'Parent');
      | next_is_outport = strcmp(get_param(next_block,'BlockType'),'Outport');
      | if (last_is_inport && next_is_outport)
      |     mo.getDialogControl('BtnMoveUp').Enabled = 'off';
      |     mo.getDialogControl('BtnMoveDown').Enabled = 'off';
      |     mo.getDialogControl('BtnEdit').Enabled = 'off';
      |     mo.getDialogControl('BtnDelete').Enabled = 'off';
      | end
      | 
      | %Refresh
      | treeValues = FailureInjectionPointHelper.getAllFmAndParamsAsTreeString(gcb);
      | mo = Simulink.Mask.get(gcb);
      | dc = mo.getDialogControl('GbFmInfo');
      | treeView = dc.getDialogControl('TreeViewFM');
      | treeView.TreeItems = {};
      | treeView.TreeItems = treeValues;
      mask DialogControl BtnRefresh Prompt: Refresh
      mask DialogControl BtnRefresh Callback:
      | set_param(gcb,'LinkStatus','none');
      | 
      | treeValues = FailureInjectionPointHelper.getAllFmAndParamsAsTreeString(gcb);
      | mo = Simulink.Mask.get(gcb);
      | dc = mo.getDialogControl('GbFmInfo');
      | treeView = dc.getDialogControl('TreeViewFM');
      | treeView.TreeItems = {};
      | treeView.TreeItems = treeValues;
      mask Display: image('icons/failure_injection_point.png','center')
  Out1 : Outport
  wires:
  In1/1 -> FG sensor shock absorber FIP2/1(In1)
  FG sensor shock absorber FIP2/1(Out1) -> Out1/1
